simulink model "publisher"  (R2019b)
settings: Solver=VariableStepAuto  StartTime=0.0  StopTime=10.0  RelTol=1e-3
settings Model: Creator=USER  LastModifiedBy=USER

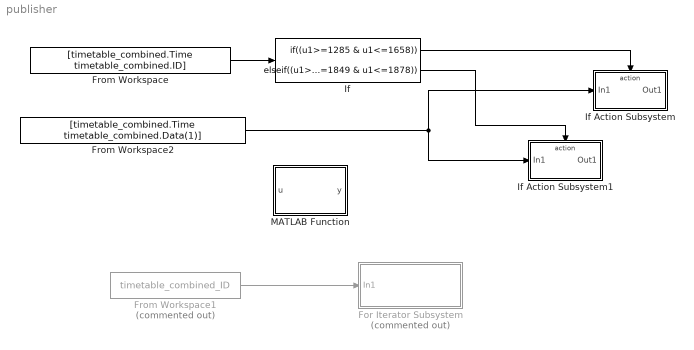
== system publisher ==
  For Iterator Subsystem : Subsystem  Commented=on  TreatAsAtomicUnit=on
  From Workspace : FromWorkspace  VariableName=[timetable_combined.Time timetable_combined.ID]  SampleTime=0
  From Workspace1 : FromWorkspace  Commented=on  VariableName=timetable_combined_ID  SampleTime=0
  From Workspace2 : FromWorkspace  VariableName=[timetable_combined.Time timetable_combined.Data(1)]  SampleTime=0
  If : If  IfExpression=(u1>=1285 & u1<=1658)  ElseIfExpressions=(u1>=1849 & u1<=1878)  ShowElse=off
  If Action Subsystem : Subsystem  TreatAsAtomicUnit=on
  If Action Subsystem1 : Subsystem  TreatAsAtomicUnit=on
  MATLAB Function : MATLAB Function  TreatAsAtomicUnit=on
  wires:
  From Workspace1/1 -> For Iterator Subsystem/1(In1)
  From Workspace/1 -> If/1
  If/1 -> If Action Subsystem/Action
  If/2 -> If Action Subsystem1/Action
  From Workspace2/1 -> If Action Subsystem1/1(In1), If Action Subsystem/1(In1)

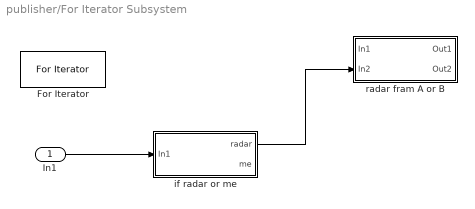
== system publisher/For Iterator Subsystem ==
  In1 : Inport
  For Iterator : ForIterator  IterationLimit=table_length
  "if radar or me " : Subsystem
  radar fram A or B : Subsystem
  wires:
  In1/1 -> "if radar or me "/1(In1)
  "if radar or me "/1(radar) -> radar fram A or B/2(In2)

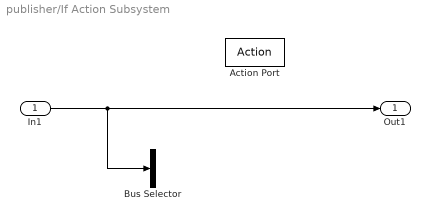
== system publisher/If Action Subsystem ==
  In1 : Inport
  Action Port : ActionPort  ActionPortLabel=if(u1 > 0)
  Bus Selector : BusSelector  OutputSignals=signal1,signal2
  Out1 : Outport
  wires:
  In1/1 -> Bus Selector/1, Out1/1

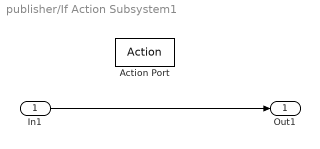
== system publisher/If Action Subsystem1 ==
  In1 : Inport
  Action Port : ActionPort  ActionPortLabel=elseif((u1>=1849 & u1<=1878))
  Out1 : Outport
  wires:
  In1/1 -> Out1/1

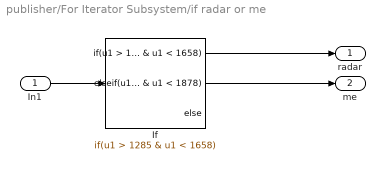
== system publisher/For Iterator Subsystem/if radar or me  ==
  In1 : Inport
  If : If  IfExpression=u1 > 1285 & u1 < 1658  ElseIfExpressions=u1 > 1849 & u1 < 1878
  radar : Outport
  me : Outport  Port=2
  wires:
  In1/1 -> If/1
  If/1 -> radar/1
  If/2 -> me/1

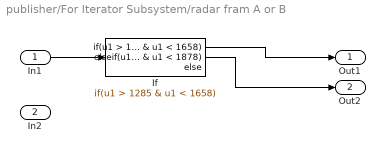
== system publisher/For Iterator Subsystem/radar fram A or B ==
  In1 : Inport
  In2 : Inport  Port=2
  If : If  IfExpression=u1 > 1285 & u1 < 1658  ElseIfExpressions=u1 > 1849 & u1 < 1878
  Out1 : Outport
  Out2 : Outport  Port=2
  wires:
  In1/1 -> If/1
  If/1 -> Out1/1
  If/2 -> Out2/1

== matlab function publisher/MATLAB Function ==
  data: u input; y output
function y = fcn(u)

y = u;
